simulink model "lab1_sim"  (R2020b)
settings: Solver=VariableStepAuto  StartTime=0.0  StopTime=10  RelTol=1e-3
settings Model: Creator=student  LastModifiedBy=student

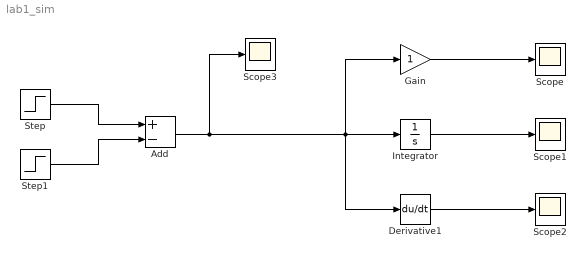
== system lab1_sim ==
  Add : Sum  Inputs=+-
  Derivative1 : Derivative
  Gain : Gain
  Integrator : Integrator
  Scope{,1..3} (4 alike) : Scope
  Step : Step  After=1000  SampleTime=0
  Step1 : Step  Time=1.005  After=1000  SampleTime=0
  wires:
  Add/1 -> Derivative1/1, Integrator/1, Gain/1, Scope3/1
  Step1/1 -> Add/2
  Step/1 -> Add/1
  Derivative1/1 -> Scope2/1
  Integrator/1 -> Scope1/1
  Gain/1 -> Scope/1
